simulink model "Insulin_Minimal_model"  (R2014a)
settings: Solver=ode3  StartTime=0.0  StopTime=180  FixedStep=0.01  RelTol=1e-3
values from neighbouring files (symbols this model uses):
  I0 = Ib + 396    (= 411)    [Modified_Bergman.m]    (also in data.m = 300)
settings Model: Creator=sameer  LastModifiedBy=sameer

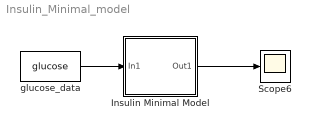
== system Insulin_Minimal_model ==
  "Insulin Minimal Model " : Subsystem
  Scope6 : Scope
      settings: SaveName=I2
  "glucose_data " : FromWorkspace  VariableName=glucose  SampleTime=0.01
  wires:
  "glucose_data "/1 -> "Insulin Minimal Model "/1(In1)
  "Insulin Minimal Model "/1(Out1) -> Scope6/1

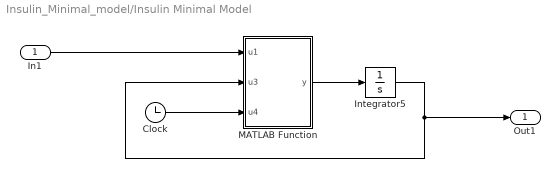
== system Insulin_Minimal_model/Insulin Minimal Model  ==
  In1 : Inport
  Clock : Clock
  Integrator5 : Integrator  InitialCondition=I0
  MATLAB Function : MATLAB Function  TreatAsAtomicUnit=on
  Out1 : Outport
  wires:
  MATLAB Function/1(y) -> Integrator5/1
  Clock/1 -> MATLAB Function/3(u4)
  Integrator5/1 -> MATLAB Function/2(u3), Out1/1
  In1/1 -> MATLAB Function/1(u1)

== matlab function Insulin_Minimal_model/Insulin Minimal Model /MATLAB Function ==
  data: u1 input; y output; u3 input; u4 input
function y  = fcn(u1,u3,u4)
p4 = 0.3;
p5 = 94;
p6 = 0.003349;
Ib = 7.3;

if(u1 - p5) > 0
    y = p6*(u1 - p5)*u4 - p4*(u3 - Ib);
else
    y = -p4*(u3 - Ib);
end
